simulink model "BlockDiagram"  (R2023a)
settings: Solver=VariableStepAuto  StartTime=0.0  StopTime=10.0  RelTol=1e-3
libraries: visionsources x1
settings Model: Creator=thaweesaktrongtirakul  LastModifiedBy=thaweesaktrongtirakul

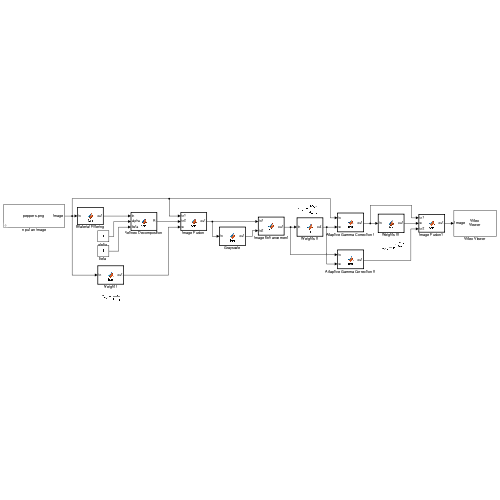
[thumbnail: Simulink's stored preview of the top-level diagram]
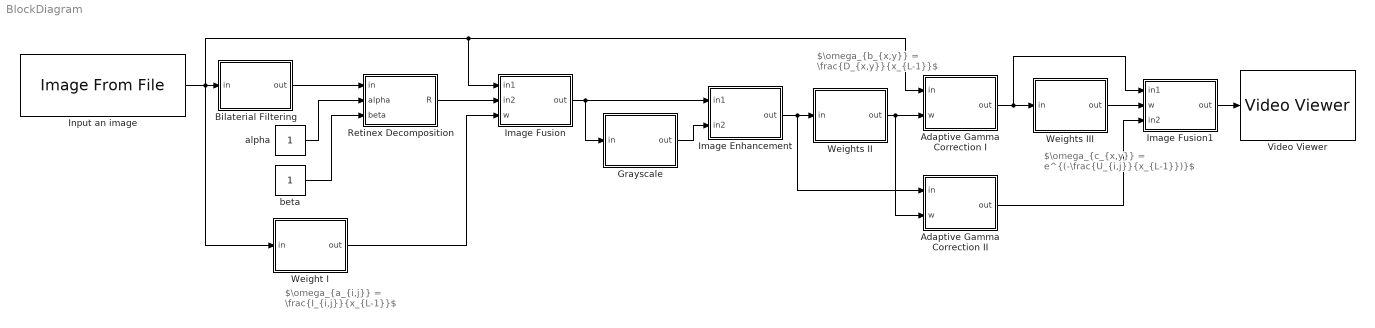
== system BlockDiagram ==
  note: $\omega_{a_{i,j}} = \frac{I_{i,j}}{x_{L-1}}$
  note: $\omega_{b_{x,y}} = \frac{D_{x,y}}{x_{L-1}}$
  note: $\omega_{c_{x,y}} = e^{(-\frac{U_{i,j}}{x_{L-1}})}$
  Adaptive Gamma Correction I : MATLAB Function  TreatAsAtomicUnit=on
  Adaptive Gamma Correction II : MATLAB Function  TreatAsAtomicUnit=on
  Bilaterial Filtering : MATLAB Function  TreatAsAtomicUnit=on
  Grayscale : MATLAB Function  TreatAsAtomicUnit=on
  Image Enhancement : MATLAB Function  TreatAsAtomicUnit=on
  Image Fusion : MATLAB Function  TreatAsAtomicUnit=on
  Image Fusion1 : MATLAB Function  TreatAsAtomicUnit=on
  Input an image : visionsources/Image From File  Tag=vipblks_nd  FileName=peppers.png  Ts=inf  imagePorts=One multidimensional signal  OutPortLabels=R|G|B  ImageDataType=Inherit from input image  sdImageDataType=uint(8)  Signed=on  WordLength=16  FractionLengthMode=User-defined  FractionLength=15
  Retinex Decomposition : MATLAB Function  TreatAsAtomicUnit=on
  Video Viewer : VideoViewer  FigPos=[2041 741 418 304]
  Weight I : MATLAB Function  TreatAsAtomicUnit=on
  Weights II : MATLAB Function  TreatAsAtomicUnit=on
  Weights III : MATLAB Function  TreatAsAtomicUnit=on
  alpha : Constant
  beta : Constant
  wires:
  Input an image/1 -> Weight I/1(in), Image Fusion/1(in1), Adaptive Gamma Correction I/1(in), Bilaterial Filtering/1(in)
  Bilaterial Filtering/1(out) -> Retinex Decomposition/1(in)
  alpha/1 -> Retinex Decomposition/2(alpha)
  beta/1 -> Retinex Decomposition/3(beta)
  Retinex Decomposition/1(R) -> Image Fusion/2(in2)
  Weight I/1(out) -> Image Fusion/3(w)
  Image Fusion/1(out) -> Grayscale/1(in), Image Enhancement/1(in1)
  Grayscale/1(out) -> Image Enhancement/2(in2)
  Image Fusion1/1(out) -> Video Viewer/1
  Weights II/1(out) -> Adaptive Gamma Correction II/2(w), Adaptive Gamma Correction I/2(w)
  Image Enhancement/1(out) -> Adaptive Gamma Correction II/1(in), Weights II/1(in)
  Adaptive Gamma Correction I/1(out) -> Image Fusion1/1(in1), Weights III/1(in)
  Weights III/1(out) -> Image Fusion1/2(w)
  Adaptive Gamma Correction II/1(out) -> Image Fusion1/3(in2)

== matlab function BlockDiagram/Bilaterial Filtering ==
  data: in input; out output
function out = fcn(in)

out = in;

== matlab function BlockDiagram/Retinex Decomposition ==
  data: in input; R output; alpha input; beta input
function R  = fcn(in,alpha,beta)

R = in;

== matlab function BlockDiagram/Image Fusion ==
  data: in1 input; out output; in2 input; w input
function out  = fcn(in1,in2,w)

out = w * in1 + (1 - w) + in2;

== matlab function BlockDiagram/Weight I ==
  data: in input; out output
function out  = fcn(in)

out = in;

== matlab function BlockDiagram/Image Enhancement ==
  data: in1 input; out output; in2 input
function out  = fcn(in1,in2)

out =in1 + in2;

== matlab function BlockDiagram/Grayscale ==
  data: in input; out output
function out  = fcn(in)

out = in;

== matlab function BlockDiagram/Adaptive Gamma Correction I ==
  data: in input; out output; w input
function out  = fcn(in,w)

out = w*in1 + in2;

== matlab function BlockDiagram/Adaptive Gamma Correction II ==
  data: in input; out output; w input
function out  = fcn(in,w)

out = w*in1 + in2;

== matlab function BlockDiagram/Image Fusion1 ==
  data: in1 input; w input; out output; in2 input
function out  = fcn(in1,w,in2)

out = w * in1 + (1 - w) + in2;

== matlab function BlockDiagram/Weights II ==
  data: in input; out output
function out  = fcn(in)

out = in;

== matlab function BlockDiagram/Weights III ==
  data: in input; out output
function out  = fcn(in)

out = in;
